simulink model "EvPassengerModel"  (R2019b)
settings: configuration reference "ConfigSetDesktopVariableStep" (kept outside this file)
undefined symbols (not defined in the file or in its folder): BattChrgCapcty, BattInitSoc, ChassisDistCg2RearAxle, ChassisVehMass, DiffAxleCompDamping, DiffAxleCompStiffness, DiffCarrierInertia, EnvGravCnst, EnvPrs, EnvTemp, FuelSpecificGrav, MtrEffSpdBpts, MtrInertia, TestScnrioCycleNum
libraries: autolibsharedcoupling x2, VsrLibDriver x1, VsrLibMdlConfig x1, VsrLibDriveCycleSrc x1, autolibdatasheetbattery x1, autolibshareddiff x1, LibWheels x1, autolibmappedmotor x1, LibPtSupervisoryCtrl x1, autolibshared x1
settings Model: DataDictionary=DdPassengerEv.sldd  EnableAccessToBaseWorkspace=off  SimulationMode=accelerator  PauseTimes=45  Creator=9bt  LastModifiedBy=4qz
settings ConfigSetRef: SourceName=ConfigSetDesktopVariableStep

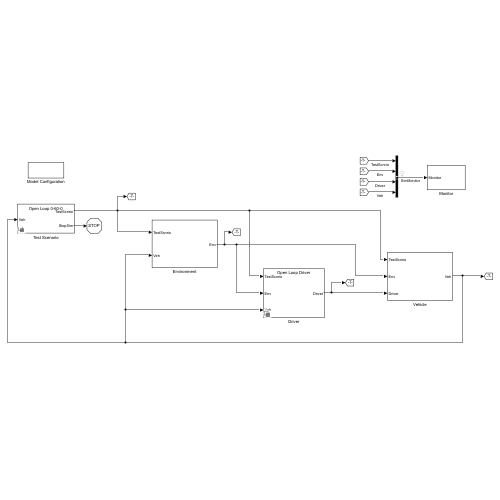
[thumbnail: Simulink's stored preview of the top-level diagram]
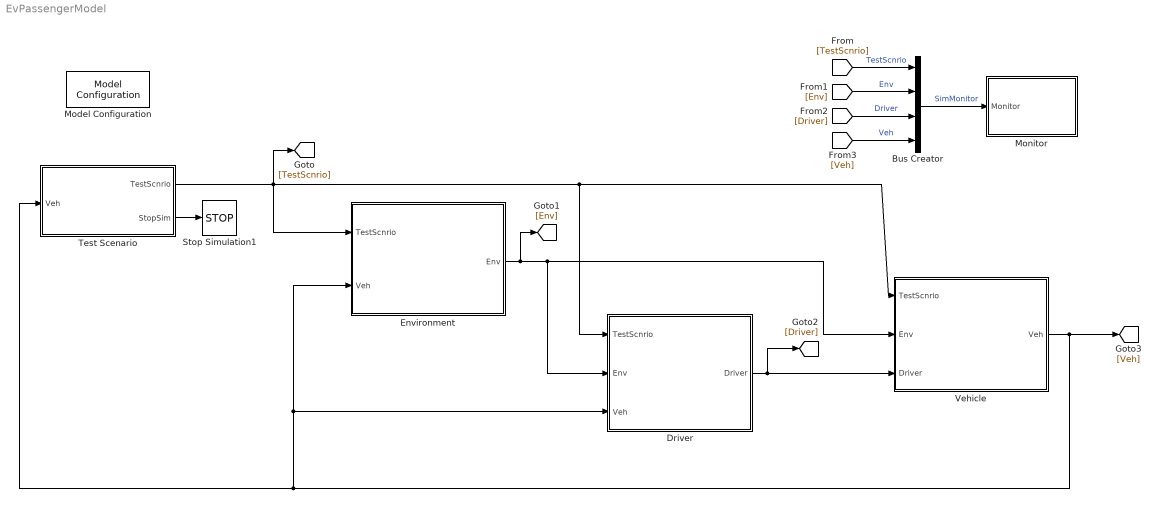
== system EvPassengerModel ==
  Bus Creator : BusCreator  Inputs=4
  Driver : Subsystem  Variant=on  VariantControlMode=label  LabelModeActiveChoice=OpenLoopDriver
  Environment : Subsystem
  Model Configuration : VsrLibMdlConfig/Model Configuration  ConfigFileName=getMdlConfigs
  Monitor : Subsystem
  Stop Simulation1 : Stop
  Test Scenario : Subsystem  Variant=on  VariantControlMode=label  LabelModeActiveChoice=OpenLoop0to60to0
  Vehicle : Subsystem
  wires:
  Driver/1(Driver) -> Vehicle/3(Driver), [Driver]
  Environment/1(Env) -> [Env], Driver/2(Env), Vehicle/2(Env)
  Test Scenario/1(TestScnrio) -> [TestScnrio], Driver/1(TestScnrio), Vehicle/1(TestScnrio), Environment/1(TestScnrio)
  Bus Creator/1 -> Monitor/1(Monitor)  "SimMonitor"
  [TestScnrio] -> Bus Creator/1  "TestScnrio"
  [Env] -> Bus Creator/2  "Env"
  [Driver] -> Bus Creator/3  "Driver"
  [Veh] -> Bus Creator/4  "Veh"
  Vehicle/1(Veh) -> [Veh], Test Scenario/1(Veh), Environment/2(Veh), Driver/3(Veh)
  Test Scenario/2(StopSim) -> Stop Simulation1/1

== system EvPassengerModel/Driver ==
  TestScnrio : Inport
  Env : Inport  Port=2
  Veh : Inport  Port=3
  Open Loop Driver : Subsystem  VariantControl=OpenLoopDriver
  Predictive Driver : Subsystem  VariantControl=PredDriver
  Driver : Outport

== system EvPassengerModel/Environment ==
  TestScnrio : Inport
  Veh : Inport  Port=2
  Subsystem : Subsystem
  Subsystem1 : Subsystem
      mask Display: disp('')
  Subsystem2 : Subsystem
      mask Display: disp('')
  Env : Outport
  wires:
  Veh/1 -> Subsystem2/2(Veh)
  Subsystem/3(WindVel) -> Subsystem1/3(WindVel)
  Subsystem/2(EnvTemp) -> Subsystem1/2(EnvTemp)
  Subsystem/4(RoadGrade) -> Subsystem1/4(RoadGrade)
  Subsystem/1(EnvPrs) -> Subsystem1/1(EnvPrs)
  Subsystem1/1(Env) -> Env/1
  TestScnrio/1 -> Subsystem2/1(TestScnrio)
  Subsystem2/1(Grade) -> Subsystem/1(Grade)

== system EvPassengerModel/Monitor ==
  Monitor : Inport
  Calculate Fuel MPG : Subsystem  Commented=on
  Calculate Powertrain Energy : Subsystem
  Terminator : Terminator
  Terminator3 : Terminator
  wires:
  Calculate Fuel MPG/1(FuelEconMPG) -> Terminator/1  "FuelEconMpg"
  Monitor/1 -> Calculate Powertrain Energy/1(Monitor), Calculate Fuel MPG/1(Monitor)
  Calculate Powertrain Energy/1(TransEnrgyOutkWh) -> Terminator3/1  "DiffEnrgyInkWh"

== system EvPassengerModel/Test Scenario ==
  Veh : Inport
  Drive Cycle Source : Subsystem  VariantControl=DriveCycleSrc
  Open Loop 0-60-0 : Subsystem  VariantControl=OpenLoop0to60to0
  TestScnrio : Outport
  StopSim : Outport  Port=2

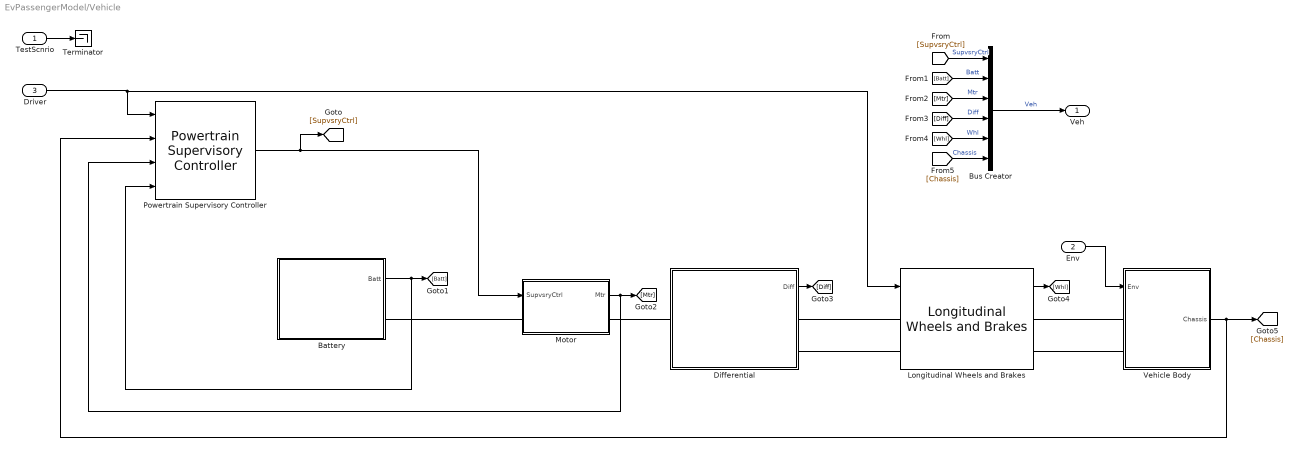
== system EvPassengerModel/Vehicle ==
  TestScnrio : Inport
  Env : Inport  Port=2
  Driver : Inport  Port=3
  Battery : Subsystem
  Bus Creator : BusCreator  Inputs=6
  Differential : Subsystem  VariantControl=0
  Longitudinal Wheels and Brakes : LibWheels/Longitudinal Wheels and Brakes  SystemSampleTime=-1  Latency=0  AutoFrameSizeCalculation=off
  Motor : Subsystem
  "Powertrain Supervisory Controller " : LibPtSupervisoryCtrl/Powertrain Supervisory Controller   SystemSampleTime=-1  Latency=0  AutoFrameSizeCalculation=off
  Terminator : Terminator
  Vehicle Body : Subsystem
  Veh : Outport
  wires:
  "Powertrain Supervisory Controller "/1 -> Motor/1(SupvsryCtrl), [SupvsryCtrl]
  Driver/1 -> Longitudinal Wheels and Brakes/1, "Powertrain Supervisory Controller "/1
  Bus Creator/1 -> Veh/1  "Veh"
  TestScnrio/1 -> Terminator/1
  Env/1 -> Vehicle Body/1(Env)
  Vehicle Body/1(Chassis) -> "Powertrain Supervisory Controller "/2, [Chassis]
  Differential/1(Diff) -> [Diff]
  Longitudinal Wheels and Brakes/1 -> [Whl]
  [SupvsryCtrl] -> Bus Creator/1  "SupvsryCtrl"
  [Batt] -> Bus Creator/2  "Batt"
  [Mtr] -> Bus Creator/3  "Mtr"
  [Diff] -> Bus Creator/4  "Diff"
  [Whl] -> Bus Creator/5  "Whl"
  [Chassis] -> Bus Creator/6  "Chassis"
  Battery/1(Batt) -> "Powertrain Supervisory Controller "/4, [Batt]
  Motor/1(Mtr) -> "Powertrain Supervisory Controller "/3, [Mtr]
  connections:
  Battery/RConn1 -- Motor/LConn1
  Differential/LConn1 -- Motor/RConn1
  Longitudinal Wheels and Brakes/LConn1 -- Differential/RConn1
  Longitudinal Wheels and Brakes/LConn2 -- Differential/RConn2
  Longitudinal Wheels and Brakes/RConn1 -- Vehicle Body/LConn1
  Longitudinal Wheels and Brakes/RConn2 -- Vehicle Body/LConn2

== system EvPassengerModel/Driver/Open Loop Driver ==
  TestScnrio : Inport
  Env : Inport  Port=2
  Veh : Inport  Port=3
  Longitudinal Driver : Subsystem
  Subsystem1 : Subsystem
      mask Display: disp('')
  Subsystem2 : Subsystem
      mask Display: disp('')
  Driver : Outport
  wires:
  Subsystem2/2(DecelCmd) -> Longitudinal Driver/2(DecelCmdIn)
  Subsystem2/1(AccelCmd) -> Longitudinal Driver/1(AccelCmdIn)
  Veh/1 -> Subsystem2/3(Veh)
  Env/1 -> Subsystem2/2(Env)
  TestScnrio/1 -> Subsystem2/1(TestScnrio)
  Subsystem1/1(TransPlant) -> Driver/1
  Longitudinal Driver/5(IgSw) -> Subsystem1/5(IgSw)
  Longitudinal Driver/1(AccelCmd) -> Subsystem1/1(AccelCmd)
  Longitudinal Driver/4(CltchCmd) -> Subsystem1/4(CltchCmd)
  Longitudinal Driver/2(DecelCmd) -> Subsystem1/2(DecelCmd)
  Longitudinal Driver/3(GearCmd) -> Subsystem1/3(GearCmd)

== system EvPassengerModel/Driver/Predictive Driver ==
  TestScnrio : Inport
  Env : Inport  Port=2
  Veh : Inport  Port=3
  Longitudinal Driver : Subsystem
  Subsystem1 : Subsystem
      mask Display: disp('')
  Subsystem2 : Subsystem
      mask Display: disp('')
  Driver : Outport
  wires:
  Longitudinal Driver/3(GearCmd) -> Subsystem1/3(GearCmd)
  Longitudinal Driver/2(DecelCmd) -> Subsystem1/2(DecelCmd)
  Longitudinal Driver/4(CltchCmd) -> Subsystem1/4(CltchCmd)
  Longitudinal Driver/1(AccelCmd) -> Subsystem1/1(AccelCmd)
  Longitudinal Driver/5(IgSw) -> Subsystem1/5(IgSw)
  Subsystem1/1(TransPlant) -> Driver/1
  TestScnrio/1 -> Subsystem2/1(TestScnrio)
  Env/1 -> Subsystem2/2(Env)
  Veh/1 -> Subsystem2/3(Veh)
  Subsystem2/1(VehRefSpd) -> Longitudinal Driver/1(VehRefSpd)
  Subsystem2/2(VehRefSpdLookAhead) -> Longitudinal Driver/2(VehRefSpdLookAhead)
  Subsystem2/3(VehDistLookAhead) -> Longitudinal Driver/3(VehDistLookAhead)
  Subsystem2/4(TimeLookAhead) -> Longitudinal Driver/4(TimeLookAhead)
  Subsystem2/5(VehSpd) -> Longitudinal Driver/5(VehSpd)
  Subsystem2/6(VehDist) -> Longitudinal Driver/6(VehDist)
  Subsystem2/7(RoadGrade) -> Longitudinal Driver/7(RoadGrade)
  Subsystem2/8(GradeLookAhead) -> Longitudinal Driver/8(GradeLookAhead)

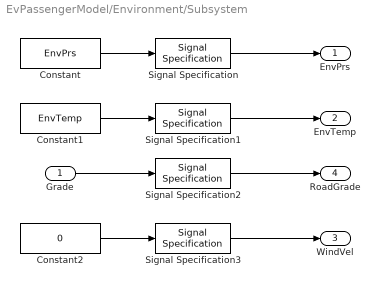
== system EvPassengerModel/Environment/Subsystem ==
  Grade : Inport
  Constant : Constant  Value=EnvPrs
  Constant1 : Constant  Value=EnvTemp
  Constant2 : Constant  Value=0
  Signal Specification : SignalSpecification  Unit=Pa
  Signal Specification1 : SignalSpecification  Unit=K
  Signal Specification2 : SignalSpecification  Unit=rad
  Signal Specification3 : SignalSpecification  Unit=m/s
  EnvPrs : Outport
  EnvTemp : Outport  Port=2
  WindVel : Outport  Port=3
  RoadGrade : Outport  Port=4
  wires:
  Constant/1 -> Signal Specification/1
  Constant2/1 -> Signal Specification3/1
  Constant1/1 -> Signal Specification1/1
  Grade/1 -> Signal Specification2/1
  Signal Specification/1 -> EnvPrs/1
  Signal Specification1/1 -> EnvTemp/1
  Signal Specification2/1 -> RoadGrade/1
  Signal Specification3/1 -> WindVel/1

== system EvPassengerModel/Environment/Subsystem1 ==
  EnvPrs : Inport
  EnvTemp : Inport  Port=2
  WindVel : Inport  Port=3
  RoadGrade : Inport  Port=4
  Bus Creator : BusCreator  Inputs=4
  Env : Outport
  wires:
  EnvPrs/1 -> Bus Creator/1  "EnvPrs"
  EnvTemp/1 -> Bus Creator/2  "EnvTemp"
  Bus Creator/1 -> Env/1  "Env"
  WindVel/1 -> Bus Creator/3  "WindVel"
  RoadGrade/1 -> Bus Creator/4  "RoadGrade"

== system EvPassengerModel/Environment/Subsystem2 ==
  TestScnrio : Inport
  Veh : Inport  Port=2
  Bus Selector : BusSelector  OutputSignals=Grade
  Terminator1 : Terminator
  Grade : Outport
  wires:
  TestScnrio/1 -> Bus Selector/1
  Bus Selector/1 -> Grade/1  "<Grade>"
  Veh/1 -> Terminator1/1

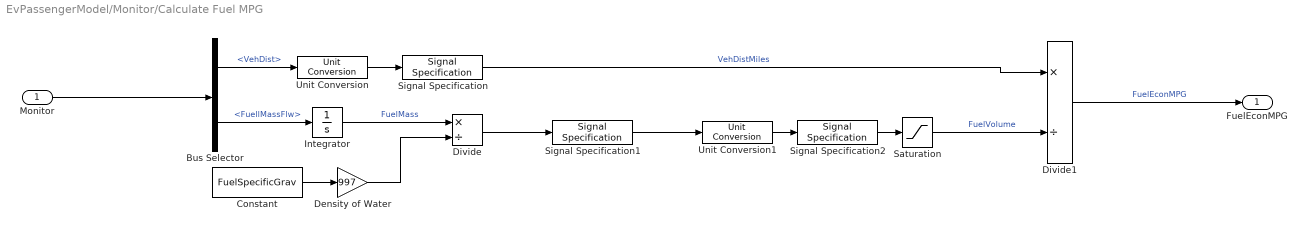
== system EvPassengerModel/Monitor/Calculate Fuel MPG ==
  Monitor : Inport
  Bus Selector : BusSelector  OutputSignals=Veh.Chassis.VehDist,Veh.Batt.EngPlant.FuellMassFlw
  Constant : Constant  Value=FuelSpecificGrav
  Density of Water : Gain  Gain=997
  Divide : Product  Inputs=*/
  Divide1 : Product  Inputs=*/
  Integrator : Integrator
  Saturation : Saturate  UpperLimit=inf  LowerLimit=1e-7
  Signal Specification : SignalSpecification  Unit=mi
  Signal Specification1 : SignalSpecification  Unit=m^3
  Signal Specification2 : SignalSpecification  Unit=gal
  Unit Conversion : UnitConversion
  Unit Conversion1 : UnitConversion
  FuelEconMPG : Outport
  wires:
  Divide1/1 -> FuelEconMPG/1  "FuelEconMPG"
  Divide/1 -> Signal Specification1/1
  Unit Conversion1/1 -> Signal Specification2/1
  Signal Specification2/1 -> Saturation/1
  Unit Conversion/1 -> Signal Specification/1
  Bus Selector/1 -> Unit Conversion/1  "<VehDist>"
  Bus Selector/2 -> Integrator/1  "<FuellMassFlw>"
  Integrator/1 -> Divide/1  "FuelMass"
  Density of Water/1 -> Divide/2
  Saturation/1 -> Divide1/2  "FuelVolume"
  Constant/1 -> Density of Water/1
  Signal Specification1/1 -> Unit Conversion1/1
  Monitor/1 -> Bus Selector/1
  Signal Specification/1 -> Divide1/1  "VehDistMiles"

== system EvPassengerModel/Monitor/Calculate Powertrain Energy ==
  Monitor : Inport
  Bus Selector2 : BusSelector  OutputSignals=Veh.Diff.PwrTrnsfrd.PwrDriveshft
  Integrator : Integrator
  Signal Specification : SignalSpecification  Unit=J
  Signal Specification1 : SignalSpecification  Unit=kW*h
  Unit Conversion : UnitConversion
  TransEnrgyOutkWh : Outport
  wires:
  Unit Conversion/1 -> Signal Specification1/1
  Integrator/1 -> Signal Specification/1  "EnrgyTrans"
  Signal Specification/1 -> Unit Conversion/1
  Signal Specification1/1 -> TransEnrgyOutkWh/1
  Monitor/1 -> Bus Selector2/1
  Bus Selector2/1 -> Integrator/1  "<PwrDriveshft>"

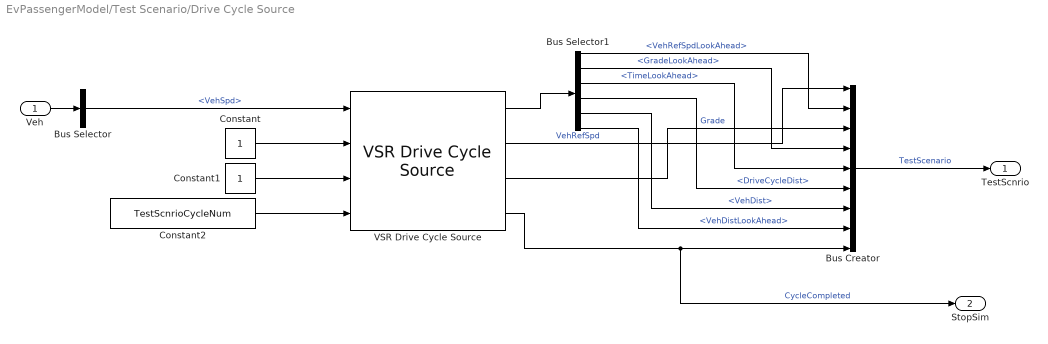
== system EvPassengerModel/Test Scenario/Drive Cycle Source ==
  Veh : Inport
  Bus Creator : BusCreator  Inputs=9
  Bus Selector : BusSelector  OutputSignals=Chassis.VehSpd
  Bus Selector1 : BusSelector  OutputSignals=VehRefSpdLookAhead,GradeLookAhead,TimeLookAhead,DriveCycleDist,VehDist,VehDistLookAhead
  Constant : Constant
  Constant1 : Constant
  Constant2 : Constant  Value=TestScnrioCycleNum
  VSR Drive Cycle Source : VsrLibDriveCycleSrc/VSR Drive Cycle Source  DistCompensationCheckbox=on  DriveCycleStructArray=TestScnrioDriveCycleStructs  TimeLookAhead=1
  TestScnrio : Outport
  StopSim : Outport  Port=2
  wires:
  VSR Drive Cycle Source/2 -> Bus Creator/1  "VehRefSpd"
  Bus Creator/1 -> TestScnrio/1  "TestScenario"
  Veh/1 -> Bus Selector/1
  VSR Drive Cycle Source/4 -> StopSim/1, Bus Creator/9  "CycleCompleted"
  VSR Drive Cycle Source/1 -> Bus Selector1/1
  Bus Selector/1 -> VSR Drive Cycle Source/1  "<VehSpd>"
  Constant/1 -> VSR Drive Cycle Source/2
  Constant1/1 -> VSR Drive Cycle Source/3
  Constant2/1 -> VSR Drive Cycle Source/4
  VSR Drive Cycle Source/3 -> Bus Creator/3  "Grade"
  Bus Selector1/1 -> Bus Creator/2  "<VehRefSpdLookAhead>"
  Bus Selector1/2 -> Bus Creator/4  "<GradeLookAhead>"
  Bus Selector1/3 -> Bus Creator/5  "<TimeLookAhead>"
  Bus Selector1/4 -> Bus Creator/6  "<DriveCycleDist>"
  Bus Selector1/6 -> Bus Creator/8  "<VehDistLookAhead>"
  Bus Selector1/5 -> Bus Creator/7  "<VehDist>"

== system EvPassengerModel/Test Scenario/Open Loop 0-60-0 ==
  Veh : Inport
  Bus Creator : BusCreator  Inputs=3
  Bus Selector : BusSelector  OutputSignals=Chassis.VehSpd
  Chart : Stateflow chart  TreatAsAtomicUnit=on
  Constant : Constant  Value=0
  Signal Specification : SignalSpecification  Unit=mph
  Unit Conversion : UnitConversion
  TestScnrio : Outport
  StopSim : Outport  Port=2
  wires:
  Bus Creator/1 -> TestScnrio/1  "TestScenario"
  Chart/1(AccelCmd) -> Bus Creator/1  "AccelCmd"
  Chart/2(DecelCmd) -> Bus Creator/2  "DecelCmd"
  Veh/1 -> Bus Selector/1
  Bus Selector/1 -> Unit Conversion/1  "<VehSpd>"
  Unit Conversion/1 -> Signal Specification/1
  Signal Specification/1 -> Chart/1(VehSpdMph)  "VehSpdMph"
  Chart/3(StopSim) -> StopSim/1
  Constant/1 -> Bus Creator/3  "Grade"

== system EvPassengerModel/Vehicle/Battery ==
  Battery : Subsystem
  Subsystem1 : Subsystem
      mask Display: disp('')
  BattOut : PMIOPort  Side=Right
  Batt : Outport
  wires:
  Battery/1(BattSoc) -> Subsystem1/1(BattSoc)
  Battery/2(BattCurr) -> Subsystem1/2(BattCurr)
  Battery/3(BattVolt) -> Subsystem1/3(BattVolt)
  Subsystem1/1(Batt) -> Batt/1
  connections:
  BattOut/RConn1 -- Battery/RConn1

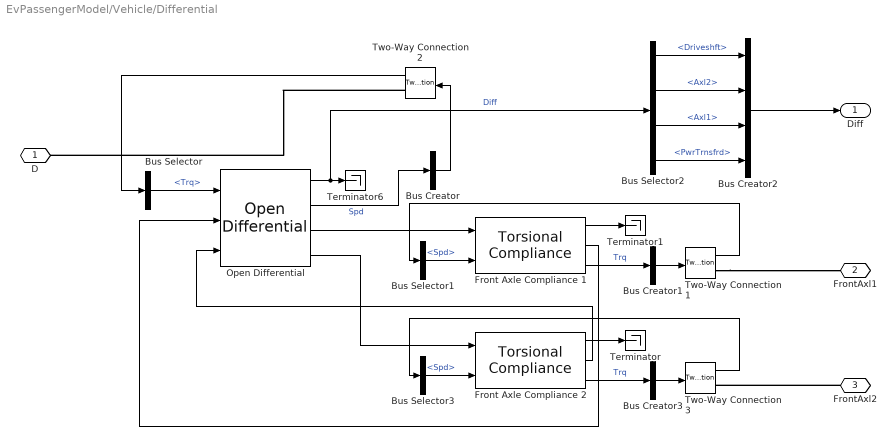
== system EvPassengerModel/Vehicle/Differential ==
  Bus Creator : BusCreator  Inputs=1
  Bus Creator1 : BusCreator  Inputs=1
  Bus Creator2 : BusCreator  Inputs=4
  Bus Creator3 : BusCreator  Inputs=1
  Bus Selector : BusSelector  OutputSignals=Trq
  Bus Selector1 : BusSelector  OutputSignals=Spd
  Bus Selector2 : BusSelector  OutputSignals=Driveshft,Axl2,Axl1,PwrInfo.PwrTrnsfrd
  Bus Selector3 : BusSelector  OutputSignals=Spd
  Front Axle Compliance 1 : autolibsharedcoupling/Torsional Compliance  port_config=Simulink  extInfo=on  k=DiffAxleCompStiffness  b=DiffAxleCompDamping  theta_o=0  domega_o=0  omega_c=DiffAxleCompCutoffFreq  blkID=0  aMode=1
  Front Axle Compliance 2 : autolibsharedcoupling/Torsional Compliance  port_config=Simulink  extInfo=on  k=DiffAxleCompStiffness  b=DiffAxleCompDamping  theta_o=0  domega_o=0  omega_c=DiffAxleCompCutoffFreq  blkID=0  aMode=1
  Open Differential : autolibshareddiff/Open Differential  DiffEffModelPopup=Constant  InterpMethod=Linear point-slope  extTamb=off  shaftSwitchMask=To the left of center-line  Ndiff=DiffRatio  Jd=DiffCarrierInertia+MtrInertia  bd=DiffCarrierDamping  Jw1=DiffAxleInertia  bw1=DiffAxleInertia  Jw2=DiffAxleInertia  bw2=DiffAxleDamping  omegaw1o=0  omegaw2o=0  eta=DiffEff  eta_tbl=reshape([0.64 0.76 0.8 0.81 0.83 0.84 0.84 0.56 0.73 0.78 0.8 0.83 0.84 0.84 0.54 0.71 0.77 0.8 0.82 0.84 0.84 0.53 0.71 0.77 0.8 0.83 0.84 0.84 0.51 0.71 0.77 0.8 0.83 0.84 0.85 0.52 0.7 0.77 0.8 0.83 0.84 0.85 0.51 0.71 0.76 0.79 0.83 0.84 0.85 0.5 0.69 0.76 0.79 0.82 0.84 0.85 0.45 0.68 0.75 0.78 0.82 0.84 0.85 0.43 0.67 0.74 0.78 0.81 0.83 0.84 0.38 0.63 0.71 0.75 0.8 0.82 0.83 0.81 0.86 0.88 0.89 0.89 0.89 0.9 0.77 0.85 0.87 0.88 0.89 0.9 0.9 0.72 0.82 0.86 0.87 0.88 0.89 0.9 0.68 0.8 0.84 0.86 0.88 0.89 0.89 0.67 0.8 0.84 0.86 0.88 0.89 0.9 0.67 0.8 0.84 0.86 0.88 0.89 0.9 0.65 0.8 0.84 0.86 0.88 0.89 0.9 0.64 0.79 0.83 0.86 0.88 0.89 0.9 0.63 0.78 0.83 0.86 0.88 0.89 0.9 0.59 0.76 0.82 0.85 0.87 0.89 0.9 0.53 0.73 0.8 0.83 0.86 0.88 0.89], 7, 11, 2)  Trq_bpts=[25, 50, 75, 100, 150, 200, 250]  omega_bpts=[52.4 78.5 105 131 157 183 209 262 314 419 524]  Temp_bpts=[290 358]  Tamb=297.15  maxAbsSpd=5e3  aMode=1
  Terminator : Terminator
  Terminator1 : Terminator
  Terminator6 : Terminator
  Two-Way Connection1 : TwoWayConnection
  Two-Way Connection2 : TwoWayConnection
  Two-Way Connection3 : TwoWayConnection
  D : PMIOPort  Side=Left
  FrontAxl1 : PMIOPort  Port=2  Side=Right
  FrontAxl2 : PMIOPort  Port=3  Side=Right
  Diff : Outport
  wires:
  Bus Creator/1 -> Two-Way Connection2/1
  Two-Way Connection2/1 -> Bus Selector/1
  Open Differential/1 -> Bus Selector2/1, Terminator6/1  "Diff"
  Open Differential/2 -> Bus Creator/1  "Spd"
  Bus Selector/1 -> Open Differential/1  "<Trq>"
  Open Differential/3 -> Front Axle Compliance 1/1
  Front Axle Compliance 1/2 -> Open Differential/2
  Front Axle Compliance 1/3 -> Bus Creator1/1  "Trq"
  Bus Creator1/1 -> Two-Way Connection1/1
  Two-Way Connection1/1 -> Bus Selector1/1
  Bus Selector1/1 -> Front Axle Compliance 1/2  "<Spd>"
  Bus Selector2/1 -> Bus Creator2/1  "<Driveshft>"
  Bus Selector2/2 -> Bus Creator2/2  "<Axl2>"
  Bus Selector2/3 -> Bus Creator2/3  "<Axl1>"
  Bus Selector2/4 -> Bus Creator2/4  "<PwrTrnsfrd>"
  Bus Creator2/1 -> Diff/1
  Bus Selector3/1 -> Front Axle Compliance 2/2  "<Spd>"
  Two-Way Connection3/1 -> Bus Selector3/1
  Bus Creator3/1 -> Two-Way Connection3/1
  Front Axle Compliance 2/3 -> Bus Creator3/1  "Trq"
  Front Axle Compliance 2/2 -> Open Differential/3
  Open Differential/4 -> Front Axle Compliance 2/1
  Front Axle Compliance 2/1 -> Terminator/1
  Front Axle Compliance 1/1 -> Terminator1/1
  connections:
  Two-Way Connection2/RConn1 -- D/RConn1
  Two-Way Connection1/RConn1 -- FrontAxl1/RConn1
  FrontAxl2/RConn1 -- Two-Way Connection3/RConn1

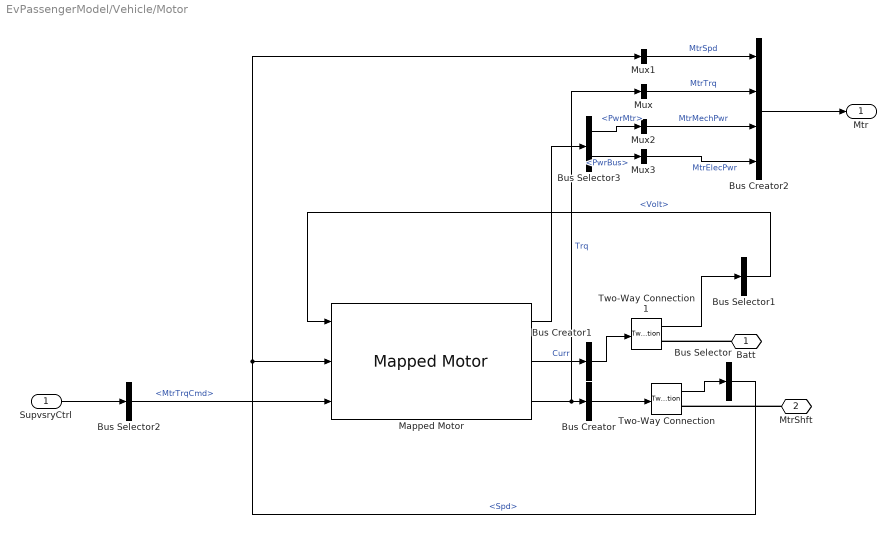
== system EvPassengerModel/Vehicle/Motor ==
  SupvsryCtrl : Inport
  Bus Creator : BusCreator  Inputs=1
  Bus Creator1 : BusCreator  Inputs=1
  Bus Creator2 : BusCreator  Inputs=4
  Bus Selector : BusSelector  OutputSignals=Spd
  Bus Selector1 : BusSelector  OutputSignals=Volt
  Bus Selector2 : BusSelector  OutputSignals=MtrTrqCmd
  Bus Selector3 : BusSelector  OutputSignals=PwrInfo.PwrTrnsfrd.PwrMtr,PwrInfo.PwrTrnsfrd.PwrBus
  Mapped Motor : autolibmappedmotor/Mapped Motor  port_config=Speed  param_by=Maximum torque and power  w_t=[ 0 375 750 800 ]  T_t=[0.09 0.08 0.07 0]  torque_max=MtrTrqMax  power_max=MtrPwrMax  Tc=MtrTrqTimeCnst  param_loss=Tabulated efficiency data  eff=100  w_eff=375  T_eff=0.08  Piron=0  Pbase=0  w_eff_bp=MtrEffSpdBpts.*pi/30  T_eff_bp=MtrEffTrqBpts  Temp_eff_bp=[233.15 293.15 373.15]  losses_table=[1 2;3 4]  losses_table_3d=cat(3,[1.49 1.67 2.21 3.10; 0.42 0.69 1.14 2.03; 0.06 0.24 0.78 1.68; 0.42 0.69 1.14 2.03; 1.49 1.67 2.21 3.10],[1.49 1.67 2.21 3.10; 0.42 0.69 1.14 2.03; 0.06 0.24 0.78 1.68; 0.42 0.69 1.14 2.03; 1.49 1.67 2.21 3.10],[1.49 1.67 2.21 3.10; 0.42 0.69 1.14 2.03; 0.06 0.24 0.78 1.68; 0.42 0.69 1.14 2.03; 1.49 1.67 2.21 3.10])  efficiency_table=MtrEffTbl  efficiency_table_3d=cat(3,[95 95 95 95; 95 95 95 95; 95 95 95 95; 95 95 95 95; 95 95 95 95],[95 95 95 95; 95 95 95 95; 95 95 95 95; 95 95 95 95; 95 95 95 95],[95 95 95 95; 95 95 95 95; 95 95 95 95; 95 95 95 95; 95 95 95 95])  J=5e-6  b=1e-5  omega_o=0  T_t_extended=[0 0.07 0.08 0.09 0.08 0.07 0]  w_t_extended=[-800 -750 -375 0 375 750 800]  KLossIron=0  KLossCopper=0  x_w_eff_vec=[-1047.1975511966 -942.477796076938 -837.758040957278 -733.038285837618 -628.318530717959 -523.598775598299 -418.879020478639 -314.159265358979 -285.714285713875 -209.43951023932 -104.71975511966 0 104.71975511966 209.43951023932 285.714285713875 314.159265358979 418.879020478639 523.598775598299 628.318530717959 733.038285837618 837.758040957278 942.477796076938 1047.1975511966]  x_T_eff_vec=[-360 -334.285714285714 -308.571428571429 -282.857142857143 -257.142857142857 -231.428571428571 -205.714285714286 -180 -154.285714285714 -128.571428571429 -102.857142857143 -77.1428571428572 -51.4285714285714 -25.7142857142857 0 25.7142857142857 51.4285714285714 77.1428571428572 102.857142857143 128.571428571429 154.285714285714 180 205.714285714286 231.428571428571 257.142857142857 282.857142857143 308.571428571429 334.285714285714 360]  x_tmp_eff_vec=[-0.09 -0.06 -0.03 0 0.03 0.06 0.09]  x_losses_mat=[28375.675580811 26348.8416107531 24322.0076406952 22295.1736706372 20268.3397005793 18241.5057305213 16214.6717604635 14187.8377904055 12161.0038203476 10134.1698502897 8107.33588023173 7024.67922541817 5983.9860068377 4751.98888778288 0 4039.19055461545 5385.58740615393 6462.70488738472 7539.82236861551 9424.7779607694 11309.7335529232 13194.6891450771 15079.644737231 16964.6003293848 18849.5559215387 20734.5115136926 22619.4671058465 24504.4226980004 26389.3782901542;21656.9365907041 20110.0125485109 18563.0885063178 17016.1644641247 15469.2404219315 13922.3163797383 12375.3923375452 10828.4682953521 9281.54425315888 7734.62021096578 6187.69616877261 4640.77212657945 3648.30114610427 4276.78999900459 0 3635.2714991539 3392.92006587697 4362.32579898468 5816.43439864625 7270.54299830782 8724.65159796934 10178.7601976309 11632.8687972925 13086.977396954 14541.0859966156 15995.1945962772 17449.3031959387 18903.4117956003 20357.5203952618;15873.3102497168 14739.502374737 13605.6944997573 12471.8866247775 11338.0787497977 10204.2708748179 9070.4629998382 7936.65512485842 6802.84724987863 5669.03937489889 4535.2314999191 4125.13077918174 3242.93435209269 3801.5911102263 0 3231.35244369236 3015.9289474462 3877.62293243083 4308.46992492315 5385.58740615394 6462.7048873847 7539.82236861549 8616.93984984629 9694.05733107705 10771.1748123078 11848.2922935386 12925.4097747694 14002.5272560002 15079.644737231;13889.1464685022 12897.0645778949 11904.9826872876 10912.9007966803 9920.81890607301 8928.7370154657 7936.65512485843 6944.57323425111 5952.4913436438 4960.40945303653 3968.32756242921 3609.48943178402 2837.5675580811 3326.39222144801 0 2827.43338823081 2638.93782901542 3392.92006587698 3769.91118430775 4712.3889803847 5654.86677646161 6597.34457253856 7539.8223686155 8482.30016469241 9424.77796076936 10367.2557568463 11309.7335529233 12252.2113490002 13194.6891450771;11904.9826872876 11054.6267810528 10204.270874818 9353.91496858314 8503.5590623483 7653.20315611346 6802.84724987865 5952.49134364381 5102.13543740897 4251.77953117417 4125.13077918174 3093.8480843863 2432.20076406951 2851.19333266973 0 2423.51433276927 2261.94671058465 2908.21719932312 3877.62293243083 4039.19055461546 4847.02866553852 5654.86677646162 6462.70488738472 7270.54299830778 8078.38110923088 8886.21922015398 9694.05733107708 10501.8954420001 11309.7335529232;9920.81890607302 9212.18898421065 8503.55906234831 7794.92914048595 7086.29921862358 6377.66929676121 5669.03937489888 4960.40945303651 4251.77953117414 3543.1496093118 3437.60898265145 2578.20673698859 2026.83397005793 2375.99444389144 0 2019.59527730772 1884.95559215387 2423.51433276927 3231.35244369236 3365.99212884621 4039.19055461544 4712.38898038468 5385.58740615393 6058.78583192315 6731.9842576924 7405.18268346165 8078.3811092309 8751.57953500012 9424.77796076937;9625.30515142404 8937.78335489375 8250.26155836348 7562.73976183318 6875.21796530288 6187.69616877259 5500.17437224232 4812.65257571202 4125.13077918173 3437.60898265146 2750.08718612116 2062.56538959087 1621.46717604634 1900.79555511315 0 1615.67622184618 1507.9644737231 1938.81146621541 2585.08195495389 3231.35244369237 3877.62293243082 4523.8934211693 5170.16390990778 5816.43439864623 6462.70488738471 7108.97537612319 7755.24586486166 8401.51635360012 9047.7868423386;12566.3706143592 11668.7727133335 10771.1748123079 9873.57691128222 7024.67922541816 6322.21130287634 5619.74338033454 4256.35133712165 3648.30114610427 3040.2509550869 2432.20076406952 2107.40376762545 1404.93584508363 1425.59666633486 0 1211.75716638463 1292.54097747694 1938.81146621542 2261.94671058465 2827.43338823082 3392.92006587697 3958.40674352314 5170.16390990778 5816.43439864623 6462.70488738471 8886.21922015399 9694.05733107709 10501.8954420002 11309.7335529233;11428.571428555 10612.2448979439 9795.91836733288 8979.5918367218 6388.64241347795 5749.77817213014 5110.91393078237 4472.04968943457 3833.18544808676 3194.32120673899 2555.45696539118 1916.59272404339 ...(+6502 chars)]  x_losses_mat_3d=[37.8947368421052 25.2631578947368 12.6315789473684 0 12 24 36;18.9473684210526 12.6315789473684 6.3157894736842 0 5.99999999999999 12 18;0 0 0 0 0 0 0;18 12 5.99999999999999 0 6.3157894736842 12.6315789473684 18.9473684210526;36 24 12 0 12.6315789473684 25.2631578947368 37.8947368421052]  CalLossMapData={}  CalLossWithTempMapData={}  aMode=aMode  RefBlkName='autolibmappedmotor/Mapped Motor'
  Mux{,1..3} (4 alike) : Mux  Inputs=1
  Two-Way Connection : TwoWayConnection
  Two-Way Connection1 : TwoWayConnection
  Batt : PMIOPort  Side=Left
  MtrShft : PMIOPort  Port=2  Side=Right
  Mtr : Outport
  wires:
  Bus Creator/1 -> Two-Way Connection/1
  Mapped Motor/3 -> Mux/1, Bus Creator/1  "Trq"
  Mapped Motor/2 -> Bus Creator1/1  "Curr"
  Bus Creator1/1 -> Two-Way Connection1/1
  Mapped Motor/1 -> Bus Selector3/1
  SupvsryCtrl/1 -> Bus Selector2/1
  Two-Way Connection/1 -> Bus Selector/1
  Two-Way Connection1/1 -> Bus Selector1/1
  Bus Selector1/1 -> Mapped Motor/1  "<Volt>"
  Bus Selector/1 -> Mux1/1, Mapped Motor/2  "<Spd>"
  Bus Selector2/1 -> Mapped Motor/3  "<MtrTrqCmd>"
  Mux/1 -> Bus Creator2/2  "MtrTrq"
  Bus Creator2/1 -> Mtr/1
  Mux2/1 -> Bus Creator2/3  "MtrMechPwr"
  Bus Selector3/1 -> Mux2/1  "<PwrMtr>"
  Mux1/1 -> Bus Creator2/1  "MtrSpd"
  Bus Selector3/2 -> Mux3/1  "<PwrBus>"
  Mux3/1 -> Bus Creator2/4  "MtrElecPwr"
  connections:
  Batt/RConn1 -- Two-Way Connection1/RConn1
  MtrShft/RConn1 -- Two-Way Connection/RConn1

== system EvPassengerModel/Vehicle/Vehicle Body ==
  Env : Inport
  Logitudinal Vehicle Body : Subsystem
  Subsystem1 : Subsystem
      mask Display: disp('')
  Subsystem4 : Subsystem
      mask Display: disp('')
  FrontAxle : PMIOPort  Side=Left
  RearDiff : PMIOPort  Port=2  Side=Left
  Chassis : Outport
  wires:
  Logitudinal Vehicle Body/1(VehSpd) -> Subsystem1/1(VehSpd)
  Logitudinal Vehicle Body/2(VehDist) -> Subsystem1/2(VehDist)
  Logitudinal Vehicle Body/3(FrontAxleFrc) -> Subsystem1/3(FrontAxleFrc)
  Logitudinal Vehicle Body/4(RearAxleFrc) -> Subsystem1/4(RearAxleFrc)
  Subsystem1/1(ChassisPlant) -> Chassis/1
  Env/1 -> Subsystem4/1(Env)
  Subsystem4/1(RoadGrade) -> Logitudinal Vehicle Body/1(RoadGrade)
  Subsystem4/2(WindVel) -> Logitudinal Vehicle Body/2(WindVel)
  connections:
  RearDiff/RConn1 -- Logitudinal Vehicle Body/LConn2
  FrontAxle/RConn1 -- Logitudinal Vehicle Body/LConn1

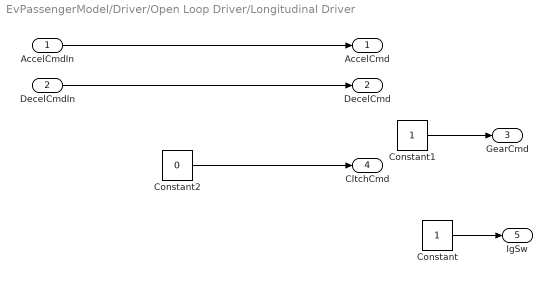
== system EvPassengerModel/Driver/Open Loop Driver/Longitudinal Driver ==
  AccelCmdIn : Inport
  DecelCmdIn : Inport  Port=2
  Constant : Constant
  Constant1 : Constant
  Constant2 : Constant  Value=0
  AccelCmd : Outport
  DecelCmd : Outport  Port=2
  GearCmd : Outport  Port=3
  CltchCmd : Outport  Port=4
  IgSw : Outport  Port=5
  wires:
  Constant1/1 -> GearCmd/1
  Constant/1 -> IgSw/1
  DecelCmdIn/1 -> DecelCmd/1
  Constant2/1 -> CltchCmd/1
  AccelCmdIn/1 -> AccelCmd/1

== system EvPassengerModel/Driver/Open Loop Driver/Subsystem1 ==
  AccelCmd : Inport
  DecelCmd : Inport  Port=2
  GearCmd : Inport  Port=3
  CltchCmd : Inport  Port=4
  IgSw : Inport  Port=5
  Bus Creator : BusCreator  Inputs=5
  TransPlant : Outport
  wires:
  IgSw/1 -> Bus Creator/5  "IgSw"
  CltchCmd/1 -> Bus Creator/4  "CltchCmd"
  GearCmd/1 -> Bus Creator/3  "GearCmd"
  Bus Creator/1 -> TransPlant/1  "Driver"
  DecelCmd/1 -> Bus Creator/2  "DecelCmd"
  AccelCmd/1 -> Bus Creator/1  "AccelCmd"

== system EvPassengerModel/Driver/Open Loop Driver/Subsystem2 ==
  TestScnrio : Inport
  Env : Inport  Port=2
  Veh : Inport  Port=3
  Bus Selector : BusSelector  OutputSignals=AccelCmd,DecelCmd
  Terminator : Terminator
  Terminator1 : Terminator
  AccelCmd : Outport
  DecelCmd : Outport  Port=2
  wires:
  Bus Selector/1 -> AccelCmd/1  "<AccelCmd>"
  TestScnrio/1 -> Bus Selector/1
  Bus Selector/2 -> DecelCmd/1  "<DecelCmd>"
  Env/1 -> Terminator/1
  Veh/1 -> Terminator1/1

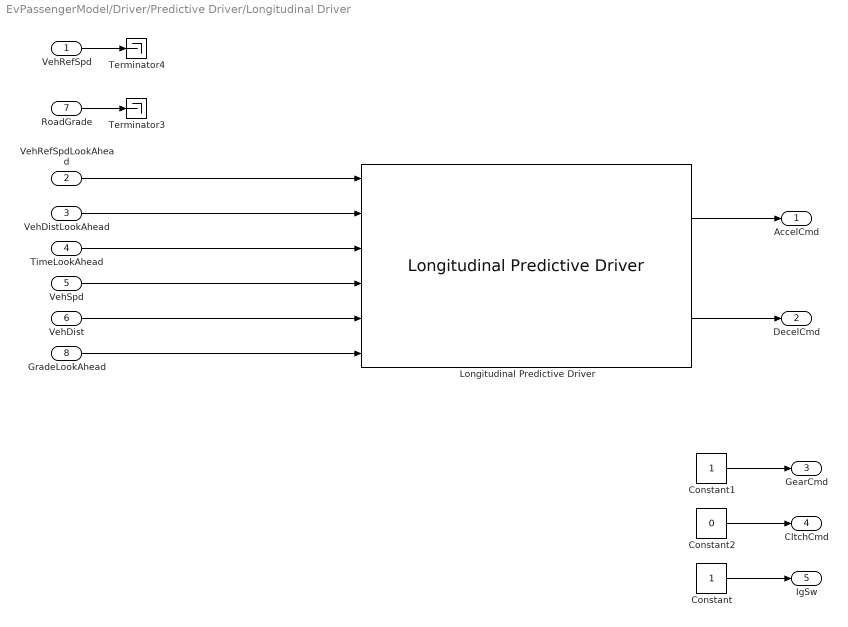
== system EvPassengerModel/Driver/Predictive Driver/Longitudinal Driver ==
  VehRefSpd : Inport
  VehRefSpdLookAhead : Inport  Port=2
  VehDistLookAhead : Inport  Port=3
  TimeLookAhead : Inport  Port=4
  VehSpd : Inport  Port=5
  VehDist : Inport  Port=6
  RoadGrade : Inport  Port=7
  GradeLookAhead : Inport  Port=8
  Constant : Constant
  Constant1 : Constant
  Constant2 : Constant  Value=0
  Longitudinal Predictive Driver : VsrLibDriver/Longitudinal Predictive Driver  VehMass=ChassisVehMass  aR=DriverLongLossA  bR=DriverLongLossB  cR=DriverLongLossC  MaxAccelFrcSpdBpts=DriverMaxAccelFrcSpdBpts  MaxAccelFrcTbl=DriverMaxAccelFrcTbl  AccelPdlBpts=DriverAccelPdlBpts  AccelPdlTbl=DriverAccelPdlTbl  BrakePdlBpts=DriverBrakePdlBpts  BrakeFrcTbl=DriverBrakeFrcTbl  SmoothTimeAvg=DriverSmoothTimeAvg  VelThresh=DriverVelThresh  PdlRateLimitWeight=DriverPdlRateLimitWeight  DistOptWeight=DriverDistOptWeight  NumOptimIters=DriverNumOptimIters  g=EnvGravCnst
  Terminator3 : Terminator
  Terminator4 : Terminator
  AccelCmd : Outport
  DecelCmd : Outport  Port=2
  GearCmd : Outport  Port=3
  CltchCmd : Outport  Port=4
  IgSw : Outport  Port=5
  wires:
  VehRefSpd/1 -> Terminator4/1
  RoadGrade/1 -> Terminator3/1
  VehSpd/1 -> Longitudinal Predictive Driver/4
  Constant/1 -> IgSw/1
  Constant1/1 -> GearCmd/1
  GradeLookAhead/1 -> Longitudinal Predictive Driver/6
  VehRefSpdLookAhead/1 -> Longitudinal Predictive Driver/1
  TimeLookAhead/1 -> Longitudinal Predictive Driver/3
  Longitudinal Predictive Driver/1 -> AccelCmd/1
  Longitudinal Predictive Driver/2 -> DecelCmd/1
  Constant2/1 -> CltchCmd/1
  VehDistLookAhead/1 -> Longitudinal Predictive Driver/2
  VehDist/1 -> Longitudinal Predictive Driver/5

== system EvPassengerModel/Driver/Predictive Driver/Subsystem1 ==
  AccelCmd : Inport
  DecelCmd : Inport  Port=2
  GearCmd : Inport  Port=3
  CltchCmd : Inport  Port=4
  IgSw : Inport  Port=5
  Bus Creator : BusCreator  Inputs=5
  TransPlant : Outport
  wires:
  AccelCmd/1 -> Bus Creator/1  "AccelCmd"
  DecelCmd/1 -> Bus Creator/2  "DecelCmd"
  Bus Creator/1 -> TransPlant/1  "Driver"
  GearCmd/1 -> Bus Creator/3  "GearCmd"
  CltchCmd/1 -> Bus Creator/4  "CltchCmd"
  IgSw/1 -> Bus Creator/5  "IgSw"

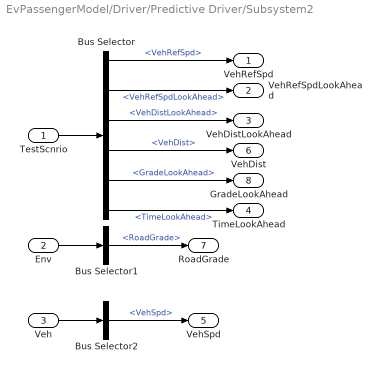
== system EvPassengerModel/Driver/Predictive Driver/Subsystem2 ==
  TestScnrio : Inport
  Env : Inport  Port=2
  Veh : Inport  Port=3
  Bus Selector : BusSelector  OutputSignals=VehRefSpd,VehRefSpdLookAhead,VehDistLookAhead,VehDist,GradeLookAhead,TimeLookAhead
  Bus Selector1 : BusSelector  OutputSignals=RoadGrade
  Bus Selector2 : BusSelector  OutputSignals=Chassis.VehSpd
  VehRefSpd : Outport
  VehRefSpdLookAhead : Outport  Port=2
  VehDistLookAhead : Outport  Port=3
  TimeLookAhead : Outport  Port=4
  VehSpd : Outport  Port=5
  VehDist : Outport  Port=6
  RoadGrade : Outport  Port=7
  GradeLookAhead : Outport  Port=8
  wires:
  TestScnrio/1 -> Bus Selector/1
  Env/1 -> Bus Selector1/1
  Bus Selector1/1 -> RoadGrade/1  "<RoadGrade>"
  Veh/1 -> Bus Selector2/1
  Bus Selector2/1 -> VehSpd/1  "<VehSpd>"
  Bus Selector/1 -> VehRefSpd/1  "<VehRefSpd>"
  Bus Selector/2 -> VehRefSpdLookAhead/1  "<VehRefSpdLookAhead>"
  Bus Selector/3 -> VehDistLookAhead/1  "<VehDistLookAhead>"
  Bus Selector/4 -> VehDist/1  "<VehDist>"
  Bus Selector/5 -> GradeLookAhead/1  "<GradeLookAhead>"
  Bus Selector/6 -> TimeLookAhead/1  "<TimeLookAhead>"

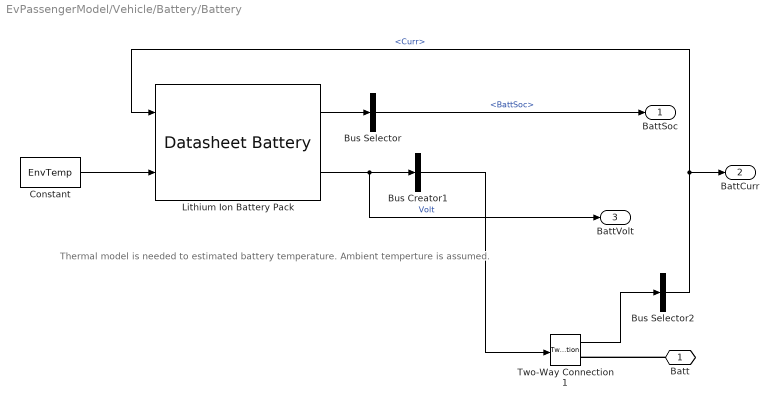
== system EvPassengerModel/Vehicle/Battery/Battery ==
  note: Thermal model is needed to estimated battery temperature. Ambient temperture is assumed.
  Bus Creator1 : BusCreator  Inputs=1
  Bus Selector : BusSelector  OutputSignals=BattSoc
  Bus Selector2 : BusSelector  OutputSignals=Curr
  Constant : Constant  Value=EnvTemp
  Lithium Ion Battery Pack : autolibdatasheetbattery/Datasheet Battery  CapacityCtrl=Parameter  OutputVlt=Unfiltered  BattChargeMax=BattChrgCapcty  Em=BattOpenVoltTbl  CapLUTBp=BattOpenVoltCapBpts  RInt=BattResistTbl  BattTempBp=BattResistTempBpts  CapSOCBp=BattResistSocBpts  Ns=BattNumCellsParallel  Np=BattNumCellsSeries  BattCapInit=BattInitSoc*BattChrgCapcty  Tc=1/1000  Vinit=3.75*72  RefBlkName='autolibdatasheetbattery/Datasheet Battery'
  Two-Way Connection1 : TwoWayConnection
  Batt : PMIOPort  Side=Right
  BattSoc : Outport
  BattCurr : Outport  Port=2  Unit=A
  BattVolt : Outport  Port=3  Unit=V
  wires:
  Bus Selector2/1 -> BattCurr/1, Lithium Ion Battery Pack/1  "<Curr>"
  Lithium Ion Battery Pack/2 -> BattVolt/1, Bus Creator1/1  "Volt"
  Bus Creator1/1 -> Two-Way Connection1/1
  Constant/1 -> Lithium Ion Battery Pack/2
  Bus Selector/1 -> BattSoc/1  "<BattSoc>"
  Lithium Ion Battery Pack/1 -> Bus Selector/1
  Two-Way Connection1/1 -> Bus Selector2/1
  connections:
  Batt/RConn1 -- Two-Way Connection1/RConn1

== system EvPassengerModel/Vehicle/Battery/Subsystem1 ==
  BattSoc : Inport
  BattCurr : Inport  Port=2
  BattVolt : Inport  Port=3
  Bus Creator : BusCreator  Inputs=3
  Batt : Outport
  wires:
  BattSoc/1 -> Bus Creator/1  "BattSoc"
  BattCurr/1 -> Bus Creator/2  "BattCurr"
  Bus Creator/1 -> Batt/1  "Batt"
  BattVolt/1 -> Bus Creator/3  "BattVolt"

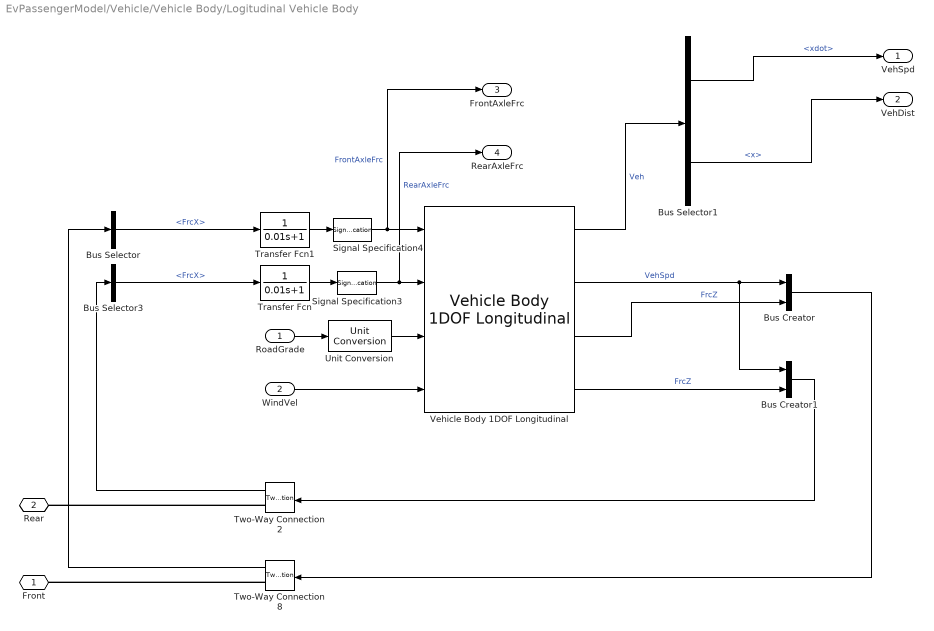
== system EvPassengerModel/Vehicle/Vehicle Body/Logitudinal Vehicle Body ==
  RoadGrade : Inport
  WindVel : Inport  Port=2  Unit=m/s
  Bus Creator : BusCreator  Inputs=2
  Bus Creator1 : BusCreator  Inputs=2
  Bus Selector : BusSelector  OutputSignals=FrcX
  Bus Selector1 : BusSelector  OutputSignals=BdyFrm.Cg.Vel.xdot,BdyFrm.Cg.Disp.x
  Bus Selector3 : BusSelector  OutputSignals=FrcX
  Signal Specification3 : SignalSpecification  Unit=N
  Signal Specification4 : SignalSpecification  Unit=N
  Transfer Fcn : TransferFcn  Denominator=[0.01 1]
  Transfer Fcn1 : TransferFcn  Denominator=[0.01 1]
  Two-Way Connection2 : TwoWayConnection
  Two-Way Connection8 : TwoWayConnection
  Unit Conversion : UnitConversion
  Vehicle Body 1DOF Longitudinal : autolibshared/Vehicle Body 1DOF Longitudinal  VariantControl=SL  extFMode=off  extMMode=off  extTamb=off  wind3D=off  aMode=1  NF=ChassisNumFrontWhls  NR=ChassisNumRearWhls  m=ChassisVehMass  a=ChassisDistCg2FrontAxle  b=ChassisDistCg2RearAxle  h=ChassisCgHeight  Cd=ChassisDragCoeff  Cl=0  Cpm=0  Af=ChassisFrontalArea  x_o=0  xdot_o=0  Pabs=EnvPrs  T=EnvTemp  g=EnvGravCnst
  Front : PMIOPort  Side=Left
  Rear : PMIOPort  Port=2  Side=Left
  VehSpd : Outport  VectorParamsAs1DForOutWhenUnconnected=off
  VehDist : Outport  Port=2  VectorParamsAs1DForOutWhenUnconnected=off
  FrontAxleFrc : Outport  Port=3  VectorParamsAs1DForOutWhenUnconnected=off
  RearAxleFrc : Outport  Port=4  VectorParamsAs1DForOutWhenUnconnected=off
  wires:
  Two-Way Connection8/1 -> Bus Selector/1
  RoadGrade/1 -> Unit Conversion/1
  Bus Selector/1 -> Transfer Fcn1/1  "<FrcX>"
  Vehicle Body 1DOF Longitudinal/2 -> Bus Creator/1, Bus Creator1/1  "VehSpd"
  Vehicle Body 1DOF Longitudinal/1 -> Bus Selector1/1  "Veh"
  Signal Specification3/1 -> RearAxleFrc/1, Vehicle Body 1DOF Longitudinal/2  "RearAxleFrc"
  Bus Creator/1 -> Two-Way Connection8/1
  Vehicle Body 1DOF Longitudinal/3 -> Bus Creator/2  "FrcZ"
  WindVel/1 -> Vehicle Body 1DOF Longitudinal/4
  Two-Way Connection2/1 -> Bus Selector3/1
  Vehicle Body 1DOF Longitudinal/4 -> Bus Creator1/2  "FrcZ"
  Bus Selector1/1 -> VehSpd/1  "<xdot>"
  Bus Selector1/2 -> VehDist/1  "<x>"
  Unit Conversion/1 -> Vehicle Body 1DOF Longitudinal/3
  Signal Specification4/1 -> FrontAxleFrc/1, Vehicle Body 1DOF Longitudinal/1  "FrontAxleFrc"
  Transfer Fcn/1 -> Signal Specification3/1
  Transfer Fcn1/1 -> Signal Specification4/1
  Bus Creator1/1 -> Two-Way Connection2/1
  Bus Selector3/1 -> Transfer Fcn/1  "<FrcX>"
  connections:
  Two-Way Connection8/RConn1 -- Front/RConn1
  Two-Way Connection2/RConn1 -- Rear/RConn1

== system EvPassengerModel/Vehicle/Vehicle Body/Subsystem1 ==
  VehSpd : Inport
  VehDist : Inport  Port=2
  FrontAxleFrc : Inport  Port=3
  RearAxleFrc : Inport  Port=4
  Bus Creator : BusCreator  Inputs=4
  ChassisPlant : Outport
  wires:
  VehSpd/1 -> Bus Creator/1  "VehSpd"
  VehDist/1 -> Bus Creator/2  "VehDist"
  Bus Creator/1 -> ChassisPlant/1  "ChassisPlant"
  FrontAxleFrc/1 -> Bus Creator/3  "FrontAxleFrc"
  RearAxleFrc/1 -> Bus Creator/4  "RearAxleFrc"

== system EvPassengerModel/Vehicle/Vehicle Body/Subsystem4 ==
  Env : Inport
  Bus Selector : BusSelector  OutputSignals=RoadGrade,WindVel
  RoadGrade : Outport  VectorParamsAs1DForOutWhenUnconnected=off
  WindVel : Outport  Port=2  VectorParamsAs1DForOutWhenUnconnected=off
  wires:
  Env/1 -> Bus Selector/1
  Bus Selector/1 -> RoadGrade/1  "<RoadGrade>"
  Bus Selector/2 -> WindVel/1  "<WindVel>"

== stateflow chart EvPassengerModel/Test Scenario/Open Loop 0-60-0/Chart ==
  state StartEngine
  state Accel
    entry:
    AccelCmd = 1;
    DecelCmd = 0;
  state Decel
    entry:
    AccelCmd = 0;
    DecelCmd = 1;
  state Hold
  state EndSim
    entry:
    StopSim = true;
  (default) -> StartEngine : {StopSim = false;
      | AccelCmd = 0;
      | DecelCmd = 1;}
  StartEngine -> Accel : [after(10,sec)]
  Decel -> Hold [order 1] : [VehSpdMph < 0.1]
  Accel -> Decel [order 1] : [VehSpdMph >= 60]
  Accel -> EndSim [order 2] : [after(100,sec)]
  Decel -> EndSim [order 2] : [after(100,sec)]
  Hold -> EndSim : [after(10,sec)]
  data: VehSpdMph input; AccelCmd output; DecelCmd output; StopSim output
